simulink model "ejercicio_A"  (R2018a)
settings: Solver=VariableStepAuto  StartTime=0.0  StopTime=10.0  RelTol=1e-3
settings Model: Creator=Jorja_000  LastModifiedBy=Jorja_000

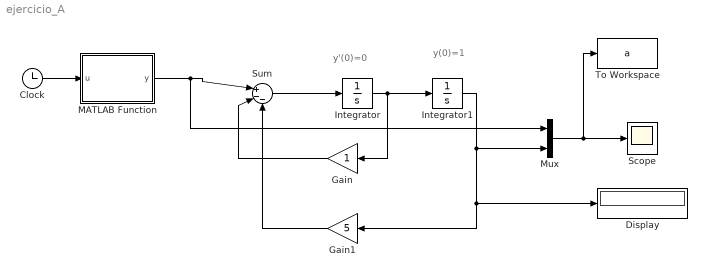
== system ejercicio_A ==
  note: y(0)=1
  note: y'(0)=0
  Clock : Clock
  Display : Display
  Gain : Gain
  Gain1 : Gain  Gain=5
  Integrator : Integrator
  Integrator1 : Integrator  InitialCondition=1
  MATLAB Function : MATLAB Function  TreatAsAtomicUnit=on
  Mux : Mux  Inputs=2
  Scope : Scope
  Sum : Sum  Inputs=|+--
  To Workspace : ToWorkspace  VariableName=a  SaveFormat=Timeseries  SampleTime=-1
  wires:
  Integrator/1 -> Gain/1, Integrator1/1
  Integrator1/1 -> Mux/2, Display/1, Gain1/1
  Gain/1 -> Sum/2
  Gain1/1 -> Sum/3
  Sum/1 -> Integrator/1
  Mux/1 -> To Workspace/1, Scope/1
  MATLAB Function/1(y) -> Mux/1, Sum/1
  Clock/1 -> MATLAB Function/1(u)

== matlab function ejercicio_A/MATLAB Function ==
  data: u input; y output
function y = fcn(u)

if(u>=0)
    y=2*cos((4*u)-pi/3);
else
    y=0;
end
